simulink model "Final_DellaVedova_SimControlador2021"  (R2021a)
settings: Solver=ode4  StartTime=0.0  StopTime=30.0  FixedStep=0.001  RelTol=1e-3
libraries: cstblocks x1
settings Model: Creator=aghersin  LastModifiedBy=maxirodriguez
settings SolverCC: AlgebraicLoopSolver=TrustRegion
settings DataIOCC: ReturnWorkspaceOutputs=off
settings OptimizationCC: LifeSpan=inf
settings DebuggingCC: SFExecutionAtInitializationDiag=none  ArithmeticOperatorsInVariantConditions=warning
settings SFSimCC: SimUseLocalCustomCode=off  CustomCodeUndefinedFunction=UseInterfaceOnly
settings RTWCC: RTWUseLocalCustomCode=off
settings CodeAppCC: StateflowObjectComments=on

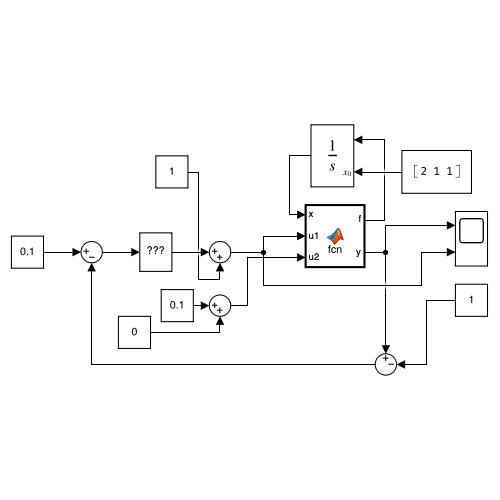
[thumbnail: Simulink's stored preview of the top-level diagram]
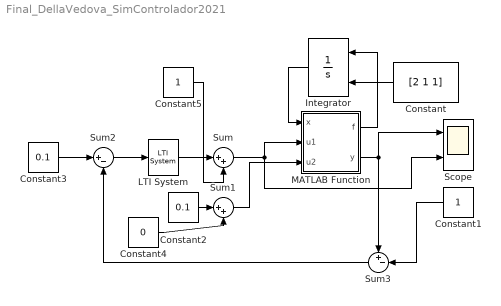
== system Final_DellaVedova_SimControlador2021 ==
  Constant : Constant  Value=[2 1 1]
  Constant1 : Constant
  Constant2 : Constant  Value=0.1
  Constant3 : Constant  Value=0.1
  Constant4 : Constant  Value=0
  Constant5 : Constant
  Integrator : Integrator  InitialConditionSource=external
  LTI System : cstblocks/LTI System  sys=Cz  IC=[]
  MATLAB Function : MATLAB Function  TreatAsAtomicUnit=on
  Scope : Scope  NumInputPorts=2
  Sum : Sum  Inputs=|++
  Sum1 : Sum  Inputs=|++
  Sum2 : Sum  Inputs=|+-
  Sum3 : Sum  Inputs=+-|
  wires:
  Integrator/1 -> MATLAB Function/1(x)
  MATLAB Function/1(f) -> Integrator/1
  Constant/1 -> Integrator/2
  MATLAB Function/2(y) -> Sum3/1, Scope/1
  Constant1/1 -> Sum3/2
  Sum2/1 -> LTI System/1
  Constant3/1 -> Sum2/1
  Sum3/1 -> Sum2/2
  Sum/1 -> Scope/2, MATLAB Function/2(u1)
  LTI System/1 -> Sum/1
  Constant2/1 -> Sum1/1
  Sum1/1 -> MATLAB Function/3(u2)
  Constant4/1 -> Sum1/2
  Constant5/1 -> Sum/2

== matlab function Final_DellaVedova_SimControlador2021/MATLAB Function ==
  data: x input; f output; y output; u1 input; u2 input
function [f,y] = fcn(x, u1, u2)

f1=(x(3) - sqrt(x(1)-x(2)))/x(1)^2;
f2=(sqrt(x(1)-x(2)) - sqrt(x(2)) + u2)/x(2)^2;
f3=0.02*(u1-x(3));

f=[f1;f2;f3];

y=x(2);
